simulink model "sim_cart_and_item"  (R2019a)
settings: Solver=VariableStepAuto  StartTime=0.0  StopTime=inf  RelTol=1e-3
values from neighbouring files (symbols this model uses):
  flag_Pitem = true    [q6_cart_and_item_sim.m]
libraries: cstblocks x3
settings Model: Creator=mm  LastModifiedBy=Ohnishi

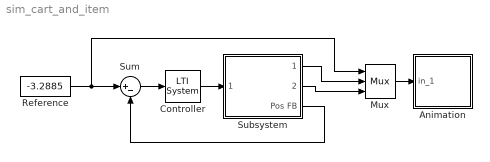
== system sim_cart_and_item ==
  Animation : Subsystem  mask(Pendulum plot){RefBlock=Reference}
      mask prompts: RefBlock "DC reference signal block name:"
      mask help: Pendulum plot
      mask Help: Pendulum animation function using Handle graphics.
      mask Display: plot([-5 -5 5 5],[0 3 3 0],[-2 -2 2 2],[0 1 1 0],[-2 -2 2 2],[1 2 2 1]);
  Controller : cstblocks/LTI System  sys=C  IC=[]
  Mux : Mux  Inputs=3
  Reference : Constant  Value=-3.2885
  Subsystem : Subsystem
  Sum : Sum  Inputs=|+-
  wires:
  Mux/1 -> Animation/1(in_1)
  Sum/1 -> Controller/1
  Reference/1 -> Mux/1, Sum/1
  Subsystem/2(Pos Item) -> Mux/3
  Controller/1 -> Subsystem/1(Force Cart)
  Subsystem/1(Pos Cart) -> Mux/2
  Subsystem/3(Pos FB) -> Sum/2

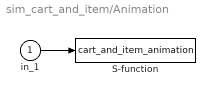
== system sim_cart_and_item/Animation ==
  in_1 : Inport
  S-function : S-Function  FunctionName=cart_and_item_animation  Parameters=RefBlock  SFunctionDeploymentMode=off  EnableBusSupport=off
      settings: DeleteFcn=pendan([],[],[],'DeleteBlock');
  wires:
  in_1/1 -> S-function/1

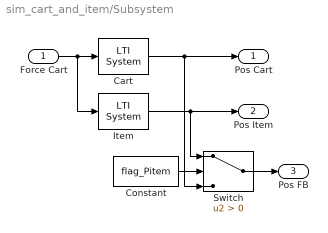
== system sim_cart_and_item/Subsystem ==
  Force Cart : Inport
  Cart : cstblocks/LTI System  sys=Pcart  IC=[]
  Constant : Constant  Value=flag_Pitem
  Item : cstblocks/LTI System  sys=Pitem  IC=[]
  Switch : Switch  Criteria=u2 > Threshold
  Pos Cart : Outport
  Pos Item : Outport  Port=2
  Pos FB : Outport  Port=3
  wires:
  Force Cart/1 -> Cart/1, Item/1
  Cart/1 -> Switch/3, Pos Cart/1
  Item/1 -> Switch/1, Pos Item/1
  Constant/1 -> Switch/2
  Switch/1 -> Pos FB/1
